simulink library "tqr"  (R2021b)
settings: Solver=VariableStepAuto  StartTime=0.0  StopTime=10.0  RelTol=1e-3
undefined symbols (not defined in the file or in its folder): ATQR_AltRDCActiveFEDUInc_X_pct, ATQR_AltRDCActiveFEDUInc_Y_enum, ATQR_AltRDCActiveFEDUTs_X_pct, ATQR_AltRDCActiveFEDUTs_Y_enum, ATQR_AltRDCActiveREDUInc_X_pct, ATQR_AltRDCActiveREDUInc_Y_enum, ATQR_AltRDCActiveREDUTs_X_pct, ATQR_AltRDCActiveREDUTs_Y_enum, ATQR_CreepFEDUTqIncSR_X_rpm, ATQR_CreepFEDUTqIncSR_Y_Nm, ATQR_CreepFEDUTs_X_rpm, ATQR_CreepFEDUTs_Y_Nm, ATQR_EcoTqFrIncGain_X_Nm, ATQR_EcoTqFrIncGain_Y_pct, ATQR_EcoTqRrIncGain_X_Nm, ATQR_EcoTqRrIncGain_Y_pct, ATQR_EL1FEDUTqDecSR_Y_Nm, ATQR_EL1FEDUTqIncSR_X_rpm, ATQR_EL1FEDUTqIncSR_Y_pct, ATQR_EL1FEDUTs_X_rpm, ATQR_EL1FEDUTs_Y_Nm, ATQR_EL1REDUTqDecSR_Y_Nm, ATQR_EL1REDUTs_Y_Nm, ATQR_FEDUEL1RegenTs_X_rpm, ATQR_FEDUTIPOutTs_X_rpm, ATQR_FrNegRateLimitIncN_X_rpm, ATQR_FrNegRateLimitIncN_Y_Nm, ATQR_FrPosRateLimitIncN_X_rpm, ATQR_FrPosRateLimitIncN_Y_Nm, ATQR_FShaftSpdTqLimCoe_X_rpm, ATQR_FTimerTqLimCoe_X_s, ATQR_FTqZeroTransUpBoundN_X_rpm, ATQR_NL1FEDUTqDecSR_Y_Nm, ATQR_NL1FEDUTqIncSR_X_rpm, ATQR_NL1FEDUTqIncSR_Y_pct, ATQR_NL1FEDUTs_X_rpm, ATQR_NL1FEDUTs_Y_Nm, ATQR_NL1REDUTqDecSR_Y_Nm, ATQR_NL1REDUTs_Y_Nm, ATQR_NormalTqFrIncGain_X_Nm, ATQR_NormalTqFrIncGain_Y_pct, ATQR_NormalTqRrIncGain_X_Nm, ATQR_NormalTqRrIncGain_Y_pct, ATQR_RrNegRateLimitIncN_X_rpm, ATQR_RrNegRateLimitIncN_Y_Nm, ATQR_RrPosRateLimitIncN_X_rpm, ATQR_RrPosRateLimitIncN_Y_Nm, ATQR_RShaftSpdTqLimCoe_X_rpm, ATQR_RTimerTqLimCoe_X_s, ATQR_SL1FEDUTqDecSR_Y_Nm, ATQR_SL1FEDUTqIncSR_X_rpm, ATQR_SL1FEDUTqIncSR_Y_pct, ATQR_SL1FEDUTs_X_rpm, ATQR_SL1FEDUTs_Y_Nm, ATQR_SL1REDUTqDecSR_Y_Nm, ATQR_SL1REDUTs_Y_Nm, ATQR_SportTqFrIncGain_X_Nm, ATQR_SportTqFrIncGain_Y_pct, ATQR_SportTqRrIncGain_X_Nm, ATQR_SportTqRrIncGain_Y_pct ... (+261)
libraries: hcu_lib x14, simulink x12, $bdroot x3
(part 5 of 9)

== system tqr/TQR/Determine Torque Request/TorqueArbitrament/TorqueSmooth/Front wheel rate limit determination/Negative Rate limit Determination ==
  VTQD_TqTargetShaftSpd_rpm : Inport
  VTQR_FEDUWhlTqReqSmoothDelay_Nm : Inport  Port=2
  VTQR_EVDriveMode_enum : Inport  Port=3
  Constant1 : Constant  Value=ENUM_DRIVEMODE_ECO
  Constant2 : Constant  Value=ENUM_DRIVEMODE_NRM
  Constant3 : Constant  Value=ENUM_DRIVEMODE_SPORT
  Constant7 : Constant  Value=ENUM_DRIVEMODE_ECO
  Constant8 : Constant  Value=ENUM_DRIVEMODE_NRM
  Constant9 : Constant  Value=ENUM_DRIVEMODE_SPORT
  Equal{1..3,5..6,8} (6 alike) : RelationalOperator  Operator===  OutDataTypeStr=boolean  RndMeth=Simplest
  If1 : If  NumInputs=3  IfExpression=u1~= 0  ElseIfExpressions=u2 ~= 0, u3 ~= 0  ShowElse=off
  If2 : If  NumInputs=3  IfExpression=u1~= 0  ElseIfExpressions=u2 ~= 0, u3 ~= 0  ShowElse=off
  Merge1 : Merge  Inputs=3
  Merge2 : Merge  Inputs=3
  Mux : Mux  Inputs=2
  VTQR_FrNegRateLimitDecE_Nm : Subsystem  TreatAsAtomicUnit=on
  VTQR_FrNegRateLimitDecN_Nm : Subsystem  TreatAsAtomicUnit=on
  VTQR_FrNegRateLimitDecS_Nm : Subsystem  TreatAsAtomicUnit=on
  VTQR_FrNegRateLimitIncE_Nm : Subsystem  TreatAsAtomicUnit=on
  VTQR_FrNegRateLimitIncN_Nm : Subsystem  TreatAsAtomicUnit=on
  VTQR_FrNegRateLimitIncS_Nm : Subsystem  TreatAsAtomicUnit=on
  VTQR_NegRateLimit_mux : Outport
  wires:
  Merge2/1 -> Mux/2  "VTQR_NegRateLimitDec_Nm"
  Constant1/1 -> Equal1/2
  [VTQD_TqTargetShaftSpd_rpm] -> VTQR_FrNegRateLimitDecE_Nm/1(VTQD_TqTargetShaftSpd_rpm)
  [VTQR_FEDUWhlTqReqSmoothDelay_Nm] -> VTQR_FrNegRateLimitDecN_Nm/2(VTQR_FEDUWhlTqReqSmoothDelay_Nm)
  [VTQD_TqTargetShaftSpd_rpm] -> VTQR_FrNegRateLimitDecN_Nm/1(VTQD_TqTargetShaftSpd_rpm)
  [VTQR_EVDriveMode_enum] -> Equal1/1
  Equal2/1 -> If2/1
  Constant2/1 -> Equal2/2
  Constant3/1 -> Equal3/2
  Equal3/1 -> If2/3
  If2/2 -> VTQR_FrNegRateLimitDecE_Nm/Action
  [VTQR_EVDriveMode_enum] -> Equal3/1
  [VTQR_EVDriveMode_enum] -> Equal2/1
  VTQR_FrNegRateLimitDecE_Nm/1(VTQR_FrNegRateLimitDecE_Nm) -> Merge2/2
  [VTQR_FEDUWhlTqReqSmoothDelay_Nm] -> VTQR_FrNegRateLimitDecE_Nm/2(VTQR_FEDUWhlTqReqSmoothDelay_Nm)
  If2/1 -> VTQR_FrNegRateLimitDecN_Nm/Action
  [VTQR_FEDUWhlTqReqSmoothDelay_Nm] -> VTQR_FrNegRateLimitDecS_Nm/2(VTQR_FEDUWhlTqReqSmoothDelay_Nm)
  [VTQD_TqTargetShaftSpd_rpm] -> VTQR_FrNegRateLimitDecS_Nm/1(VTQD_TqTargetShaftSpd_rpm)
  VTQR_FrNegRateLimitDecS_Nm/1(VTQR_FrNegRateLimitDecS_Nm) -> Merge2/3
  Equal1/1 -> If2/2
  If2/3 -> VTQR_FrNegRateLimitDecS_Nm/Action
  VTQR_FrNegRateLimitDecN_Nm/1(VTQR_FrNegRateLimitDecN_Nm) -> Merge2/1
  VTQR_FrNegRateLimitIncE_Nm/1(VTQR_FrNegRateLimitIncE_Nm) -> Merge1/2
  VTQR_FrNegRateLimitIncS_Nm/1(VTQR_FrNegRateLimitIncS_Nm) -> Merge1/3
  If1/2 -> VTQR_FrNegRateLimitIncE_Nm/Action
  If1/3 -> VTQR_FrNegRateLimitIncS_Nm/Action
  [VTQD_TqTargetShaftSpd_rpm] -> VTQR_FrNegRateLimitIncS_Nm/1(VTQD_TqTargetShaftSpd_rpm)
  [VTQR_FEDUWhlTqReqSmoothDelay_Nm] -> VTQR_FrNegRateLimitIncS_Nm/2(VTQR_FEDUWhlTqReqSmoothDelay_Nm)
  [VTQR_FEDUWhlTqReqSmoothDelay_Nm] -> VTQR_FrNegRateLimitIncE_Nm/2(VTQR_FEDUWhlTqReqSmoothDelay_Nm)
  [VTQD_TqTargetShaftSpd_rpm] -> VTQR_FrNegRateLimitIncE_Nm/1(VTQD_TqTargetShaftSpd_rpm)
  VTQR_FrNegRateLimitIncN_Nm/1(VTQR_FrNegRateLimitIncN_Nm) -> Merge1/1
  If1/1 -> VTQR_FrNegRateLimitIncN_Nm/Action
  [VTQR_FEDUWhlTqReqSmoothDelay_Nm] -> VTQR_FrNegRateLimitIncN_Nm/2(VTQR_FEDUWhlTqReqSmoothDelay_Nm)
  [VTQD_TqTargetShaftSpd_rpm] -> VTQR_FrNegRateLimitIncN_Nm/1(VTQD_TqTargetShaftSpd_rpm)
  Equal8/1 -> If1/3
  Equal5/1 -> If1/2
  Equal6/1 -> If1/1
  [VTQR_EVDriveMode_enum] -> Equal6/1
  [VTQR_EVDriveMode_enum] -> Equal8/1
  [VTQR_EVDriveMode_enum] -> Equal5/1
  Constant8/1 -> Equal6/2
  Constant9/1 -> Equal8/2
  Constant7/1 -> Equal5/2
  Merge1/1 -> Mux/1  "VTQR_NegRateLimitInc_Nm"
  Mux/1 -> VTQR_NegRateLimit_mux/1  "VTQR_NegRateLimit_mux"
  VTQD_TqTargetShaftSpd_rpm/1 -> [VTQD_TqTargetShaftSpd_rpm]
  VTQR_FEDUWhlTqReqSmoothDelay_Nm/1 -> [VTQR_FEDUWhlTqReqSmoothDelay_Nm]
  VTQR_EVDriveMode_enum/1 -> [VTQR_EVDriveMode_enum]

== system tqr/TQR/Determine Torque Request/TorqueArbitrament/TorqueSmooth/Front wheel rate limit determination/Positive Rate limit Determination ==
  VTQD_TqTargetShaftSpd_rpm : Inport
  VTQR_FEDUWhlTqReqSmoothDelay_Nm : Inport  Port=2
  VTQR_EVDriveMode_enum : Inport  Port=3
  Constant1 : Constant  Value=ENUM_DRIVEMODE_ECO
  Constant2 : Constant  Value=ENUM_DRIVEMODE_NRM
  Constant3 : Constant  Value=ENUM_DRIVEMODE_SPORT
  Constant7 : Constant  Value=ENUM_DRIVEMODE_ECO
  Constant8 : Constant  Value=ENUM_DRIVEMODE_NRM
  Constant9 : Constant  Value=ENUM_DRIVEMODE_SPORT
  Equal{1..3,5..6,8} (6 alike) : RelationalOperator  Operator===  OutDataTypeStr=boolean  RndMeth=Simplest
  If1 : If  NumInputs=3  IfExpression=u1~= 0  ElseIfExpressions=u2 ~= 0, u3 ~= 0  ShowElse=off
  If2 : If  NumInputs=3  IfExpression=u1~= 0  ElseIfExpressions=u2 ~= 0, u3 ~= 0  ShowElse=off
  Merge1 : Merge  Inputs=3
  Merge2 : Merge  Inputs=3
  Mux : Mux  Inputs=2
  VTQR_FrPosRateLimitDecE_Nm : Subsystem  TreatAsAtomicUnit=on
  VTQR_FrPosRateLimitDecN_Nm : Subsystem  TreatAsAtomicUnit=on
  VTQR_FrPosRateLimitDecS_Nm : Subsystem  TreatAsAtomicUnit=on
  VTQR_FrPosRateLimitIncE_Nm : Subsystem  TreatAsAtomicUnit=on
  VTQR_FrPosRateLimitIncN_Nm : Subsystem  TreatAsAtomicUnit=on
  VTQR_FrPosRateLimitIncS_Nm : Subsystem  TreatAsAtomicUnit=on
  VTQR_PosRateLimit_mux : Outport
  wires:
  VTQD_TqTargetShaftSpd_rpm/1 -> [VTQD_TqTargetShaftSpd_rpm]
  Mux/1 -> VTQR_PosRateLimit_mux/1  "VTQR_PosRateLimit_mux"
  Merge1/1 -> Mux/1  "VTQR_PosRateLimitInc_Nm"
  Constant7/1 -> Equal5/2
  Constant9/1 -> Equal8/2
  Constant8/1 -> Equal6/2
  [VTQR_EVDriveMode_enum] -> Equal5/1
  [VTQR_EVDriveMode_enum] -> Equal8/1
  [VTQR_EVDriveMode_enum] -> Equal6/1
  Equal6/1 -> If1/1
  Equal5/1 -> If1/2
  Equal8/1 -> If1/3
  [VTQD_TqTargetShaftSpd_rpm] -> VTQR_FrPosRateLimitIncN_Nm/1(VTQD_TqTargetShaftSpd_rpm)
  [VTQR_FEDUWhlTqReqSmoothDelay_Nm] -> VTQR_FrPosRateLimitIncN_Nm/2(VTQR_FEDUWhlTqReqSmoothDelay_Nm)
  If1/1 -> VTQR_FrPosRateLimitIncN_Nm/Action
  VTQR_FrPosRateLimitIncN_Nm/1(VTQR_FrPosRateLimitIncN_Nm) -> Merge1/1
  [VTQD_TqTargetShaftSpd_rpm] -> VTQR_FrPosRateLimitIncE_Nm/1(VTQD_TqTargetShaftSpd_rpm)
  [VTQR_FEDUWhlTqReqSmoothDelay_Nm] -> VTQR_FrPosRateLimitIncE_Nm/2(VTQR_FEDUWhlTqReqSmoothDelay_Nm)
  [VTQR_FEDUWhlTqReqSmoothDelay_Nm] -> VTQR_FrPosRateLimitIncS_Nm/2(VTQR_FEDUWhlTqReqSmoothDelay_Nm)
  [VTQD_TqTargetShaftSpd_rpm] -> VTQR_FrPosRateLimitIncS_Nm/1(VTQD_TqTargetShaftSpd_rpm)
  If1/3 -> VTQR_FrPosRateLimitIncS_Nm/Action
  If1/2 -> VTQR_FrPosRateLimitIncE_Nm/Action
  VTQR_FrPosRateLimitIncS_Nm/1(VTQR_FrPosRateLimitIncS_Nm) -> Merge1/3
  VTQR_FrPosRateLimitIncE_Nm/1(VTQR_FrPosRateLimitIncE_Nm) -> Merge1/2
  VTQR_FrPosRateLimitDecN_Nm/1(VTQR_FrPosRateLimitDecN_Nm) -> Merge2/1
  If2/3 -> VTQR_FrPosRateLimitDecS_Nm/Action
  Equal1/1 -> If2/2
  VTQR_FrPosRateLimitDecS_Nm/1(VTQR_FrPosRateLimitDecS_Nm) -> Merge2/3
  [VTQD_TqTargetShaftSpd_rpm] -> VTQR_FrPosRateLimitDecS_Nm/1(VTQD_TqTargetShaftSpd_rpm)
  [VTQR_FEDUWhlTqReqSmoothDelay_Nm] -> VTQR_FrPosRateLimitDecS_Nm/2(VTQR_FEDUWhlTqReqSmoothDelay_Nm)
  If2/1 -> VTQR_FrPosRateLimitDecN_Nm/Action
  [VTQR_FEDUWhlTqReqSmoothDelay_Nm] -> VTQR_FrPosRateLimitDecE_Nm/2(VTQR_FEDUWhlTqReqSmoothDelay_Nm)
  VTQR_FrPosRateLimitDecE_Nm/1(VTQR_FrPosRateLimitDecE_Nm) -> Merge2/2
  [VTQR_EVDriveMode_enum] -> Equal2/1
  [VTQR_EVDriveMode_enum] -> Equal3/1
  If2/2 -> VTQR_FrPosRateLimitDecE_Nm/Action
  Equal3/1 -> If2/3
  Constant3/1 -> Equal3/2
  Constant2/1 -> Equal2/2
  Equal2/1 -> If2/1
  [VTQR_EVDriveMode_enum] -> Equal1/1
  [VTQD_TqTargetShaftSpd_rpm] -> VTQR_FrPosRateLimitDecN_Nm/1(VTQD_TqTargetShaftSpd_rpm)
  [VTQR_FEDUWhlTqReqSmoothDelay_Nm] -> VTQR_FrPosRateLimitDecN_Nm/2(VTQR_FEDUWhlTqReqSmoothDelay_Nm)
  [VTQD_TqTargetShaftSpd_rpm] -> VTQR_FrPosRateLimitDecE_Nm/1(VTQD_TqTargetShaftSpd_rpm)
  Constant1/1 -> Equal1/2
  Merge2/1 -> Mux/2  "VTQR_PosRateLimitDec_Nm"
  VTQR_FEDUWhlTqReqSmoothDelay_Nm/1 -> [VTQR_FEDUWhlTqReqSmoothDelay_Nm]
  VTQR_EVDriveMode_enum/1 -> [VTQR_EVDriveMode_enum]

== system tqr/TQR/Determine Torque Request/TorqueArbitrament/TorqueSmooth/Front wheel rate limit determination/VTQR_ECOFEDURateLimitDec_Nm ==
  VTQR_FEDUWhlTqReqSmoothDelay_Nm : Inport
  VTQD_TqTargetShaftSpd_rpm : Inport  Port=2
  VTQD_RegenMode_enum : Inport  Port=3
  Action Port : ActionPort
  Constant : Constant  Value=ENUM_REGENLEVEL_LV1
  Constant1 : Constant  Value=ENUM_REGENLEVEL_LV2
  Constant2 : Constant  Value=ENUM_REGENLEVEL_LV3
  Constant3 : Constant  Value=ENUM_REGENLEVEL_LV4
  Constant4 : Constant  Value=ENUM_REGENLEVEL_LV5
  Constant5 : Constant  Value=ENUM_REGENLEVEL_OPD
  Equal{,1..5} (6 alike) : RelationalOperator  Operator===  OutDataTypeStr=boolean  RndMeth=Simplest
  If : If  NumInputs=6  IfExpression=u1~= 0  ElseIfExpressions=u2 ~= 0, u3 ~= 0,u4 ~= 0,u5~=0,u6~=0
  Invalid : Subsystem  TreatAsAtomicUnit=on
  LV1 : Subsystem  TreatAsAtomicUnit=on
  LV2 : Subsystem  AncestorBlock=tqr/TQR/Determine Torque Request/TorqueArbitrament/TorqueSmooth/Front First order filter input tau map and determination/VTQR_ECOFEDUTs_c/LV2  TreatAsAtomicUnit=on
  LV3 : Subsystem  AncestorBlock=tqr/TQR/Determine Torque Request/TorqueArbitrament/TorqueSmooth/Front First order filter input tau map and determination/VTQR_ECOFEDUTs_c/LV3  TreatAsAtomicUnit=on
  LV4 : Subsystem  AncestorBlock=tqr/TQR/Determine Torque Request/TorqueArbitrament/TorqueSmooth/Front First order filter input tau map and determination/VTQR_ECOFEDUTs_c/LV4  TreatAsAtomicUnit=on
  LV5 : Subsystem  AncestorBlock=tqr/TQR/Determine Torque Request/TorqueArbitrament/TorqueSmooth/Front First order filter input tau map and determination/VTQR_ECOFEDUTs_c/LV5  TreatAsAtomicUnit=on
  Merge : Merge  Inputs=7
  OPD : Subsystem  AncestorBlock=tqr/TQR/Determine Torque Request/TorqueArbitrament/TorqueSmooth/Front First order filter input tau map and determination/VTQR_ECOFEDUTs_c/OPD  TreatAsAtomicUnit=on
  VTQR_ECOFEDURateLimitDec_Nm : Outport
  wires:
  [VTQD_TqTargetShaftSpd_rpm] -> LV2/2(VTQD_TqTargetShaftSpd_rpm)
  Constant3/1 -> Equal3/2
  If/3 -> LV3/Action
  Equal2/1 -> If/3
  Constant4/1 -> Equal4/2
  Constant/1 -> Equal/2
  Equal5/1 -> If/6
  OPD/1(VTQR_EOPDFEDUTqDecSR_Nm) -> Merge/6
  [VTQD_RegenMode_enum] -> Equal4/1
  [VTQR_FEDUWhlTqReqSmoothDelay_Nm] -> LV2/1(VTQR_FEDUWhlTqReqSmoothDelay_Nm)
  LV2/1(VTQR_EL2FEDUTqDecSR_Nm) -> Merge/2
  [VTQD_RegenMode_enum] -> Equal5/1
  [VTQR_FEDUWhlTqReqSmoothDelay_Nm] -> OPD/1(VTQR_FEDUWhlTqReqSmoothDelay_Nm)
  [VTQD_RegenMode_enum] -> Equal2/1
  [VTQD_TqTargetShaftSpd_rpm] -> LV1/2(VTQD_TqTargetShaftSpd_rpm)
  [VTQR_FEDUWhlTqReqSmoothDelay_Nm] -> LV5/1(VTQR_FEDUWhlTqReqSmoothDelay_Nm)
  [VTQD_TqTargetShaftSpd_rpm] -> OPD/2(VTQD_TqTargetShaftSpd_rpm)
  [VTQD_TqTargetShaftSpd_rpm] -> LV4/2(VTQD_TqTargetShaftSpd_rpm)
  [VTQR_FEDUWhlTqReqSmoothDelay_Nm] -> LV3/1(VTQR_FEDUWhlTqReqSmoothDelay_Nm)
  Constant5/1 -> Equal5/2
  [VTQR_FEDUWhlTqReqSmoothDelay_Nm] -> LV4/1(VTQR_FEDUWhlTqReqSmoothDelay_Nm)
  [VTQD_TqTargetShaftSpd_rpm] -> LV5/2(VTQD_TqTargetShaftSpd_rpm)
  Equal/1 -> If/1
  If/2 -> LV2/Action
  If/4 -> LV4/Action
  Constant1/1 -> Equal1/2
  LV1/1(VTQR_EL1FEDUTqDecSR_Nm) -> Merge/1
  [VTQD_RegenMode_enum] -> Equal/1
  Equal4/1 -> If/5
  Equal1/1 -> If/2
  If/6 -> OPD/Action
  [VTQD_RegenMode_enum] -> Equal3/1
  LV3/1(VTQR_EL3FEDUTqDecSR_Nm) -> Merge/3
  LV5/1(VTQR_EL5FEDUTqIDecSR_Nm) -> Merge/5
  [VTQD_RegenMode_enum] -> Equal1/1
  Equal3/1 -> If/4
  LV4/1(VTQR_EL4FEDUTqDecSR_Nm) -> Merge/4
  [VTQD_TqTargetShaftSpd_rpm] -> LV3/2(VTQD_TqTargetShaftSpd_rpm)
  [VTQR_FEDUWhlTqReqSmoothDelay_Nm] -> LV1/1(VTQR_FEDUWhlTqReqSmoothDelay_Nm)
  If/5 -> LV5/Action
  If/1 -> LV1/Action
  Constant2/1 -> Equal2/2
  Merge/1 -> VTQR_ECOFEDURateLimitDec_Nm/1  "VTQR_ECOFEDURateLimitDec_Nm"
  VTQR_FEDUWhlTqReqSmoothDelay_Nm/1 -> [VTQR_FEDUWhlTqReqSmoothDelay_Nm]
  VTQD_TqTargetShaftSpd_rpm/1 -> [VTQD_TqTargetShaftSpd_rpm]
  VTQD_RegenMode_enum/1 -> [VTQD_RegenMode_enum]
  [VTQR_FEDUWhlTqReqSmoothDelay_Nm] -> Invalid/1(VTQR_FEDUWhlTqReqSmoothDelay_Nm)
  [VTQD_TqTargetShaftSpd_rpm] -> Invalid/2(VTQD_TqTargetShaftSpd_rpm)
  If/7 -> Invalid/Action
  Invalid/1(VTQR_EL1FEDUTqDecSR_Nm) -> Merge/7

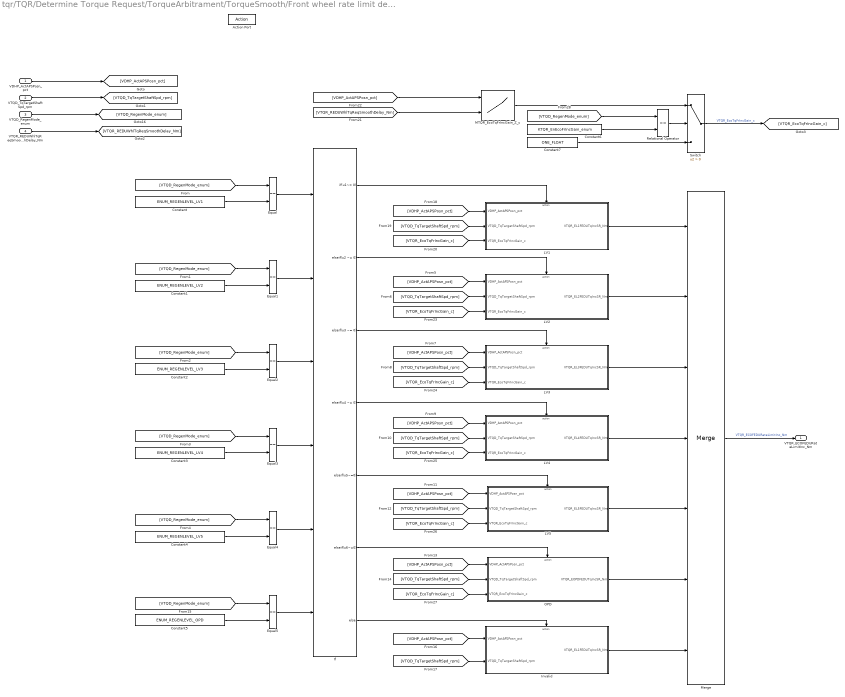
== system tqr/TQR/Determine Torque Request/TorqueArbitrament/TorqueSmooth/Front wheel rate limit determination/VTQR_ECOFEDURateLimitInc_Nm ==
  VDHP_ActAPSPosn_pct : Inport
  VTQD_TqTargetShaftSpd_rpm : Inport  Port=2
  VTQD_RegenMode_enum : Inport  Port=3
  VTQR_REDUWhlTqReqSmoothDelay_Nm : Inport  Port=4
  Action Port : ActionPort
  Constant : Constant  Value=ENUM_REGENLEVEL_LV1
  Constant1 : Constant  Value=ENUM_REGENLEVEL_LV2
  Constant2 : Constant  Value=ENUM_REGENLEVEL_LV3
  Constant3 : Constant  Value=ENUM_REGENLEVEL_LV4
  Constant4 : Constant  Value=ENUM_REGENLEVEL_LV5
  Constant5 : Constant  Value=ENUM_REGENLEVEL_OPD
  Constant6 : Constant  Value=KTQR_EnEcoFrIncGain_enum
  Constant7 : Constant  Value=ONE_FLOAT
  Equal{,1..5} (6 alike) : RelationalOperator  Operator===  OutDataTypeStr=boolean  RndMeth=Simplest
  If : If  NumInputs=6  IfExpression=u1~= 0  ElseIfExpressions=u2 ~= 0, u3 ~= 0,u4 ~= 0,u5~=0,u6~=0
  Invalid : Subsystem  TreatAsAtomicUnit=on
  LV1 : Subsystem  TreatAsAtomicUnit=on
  LV2 : Subsystem  TreatAsAtomicUnit=on
  LV3 : Subsystem  TreatAsAtomicUnit=on
  LV4 : Subsystem  TreatAsAtomicUnit=on
  LV5 : Subsystem  TreatAsAtomicUnit=on
  MTQR_EcoTqFrIncGain_Z_c : Lookup_n-D  BreakpointsForDimension1=ATQR_EcoTqFrIncGain_Y_pct  BreakpointsForDimension2=ATQR_EcoTqFrIncGain_X_Nm  Table=MTQR_EcoTqFrIncGain_Z_c  ExtrapMethod=Clip  InternalRulePriority=Speed  RndMeth=Simplest  InputSameDT=on
      settings: InputPortMap=u0,u1
  Merge : Merge  Inputs=7
  OPD : Subsystem  TreatAsAtomicUnit=on
  Relational Operator : RelationalOperator  OutDataTypeStr=boolean  RndMeth=Simplest
  Switch : Switch  Criteria=u2 > Threshold
  VTQR_ECOFEDURateLimitInc_Nm : Outport
  wires:
  [VTQD_TqTargetShaftSpd_rpm] -> LV2/2(VTQD_TqTargetShaftSpd_rpm)
  Constant3/1 -> Equal3/2
  If/3 -> LV3/Action
  Equal2/1 -> If/3
  Constant4/1 -> Equal4/2
  Constant/1 -> Equal/2
  Equal5/1 -> If/6
  OPD/1(VTQR_EOPDFEDUTqIncSR_Nm) -> Merge/6
  [VTQD_RegenMode_enum] -> Equal4/1
  [VDHP_ActAPSPosn_pct] -> LV2/1(VDHP_ActAPSPosn_pct)
  LV2/1(VTQR_EL2FEDUTqIncSR_Nm) -> Merge/2
  [VTQD_RegenMode_enum] -> Equal5/1
  [VDHP_ActAPSPosn_pct] -> OPD/1(VDHP_ActAPSPosn_pct)
  [VTQD_RegenMode_enum] -> Equal2/1
  [VTQD_TqTargetShaftSpd_rpm] -> LV1/2(VTQD_TqTargetShaftSpd_rpm)
  [VDHP_ActAPSPosn_pct] -> LV5/1(VDHP_ActAPSPosn_pct)
  [VTQD_TqTargetShaftSpd_rpm] -> OPD/2(VTQD_TqTargetShaftSpd_rpm)
  [VTQD_TqTargetShaftSpd_rpm] -> LV4/2(VTQD_TqTargetShaftSpd_rpm)
  [VDHP_ActAPSPosn_pct] -> LV3/1(VDHP_ActAPSPosn_pct)
  Constant5/1 -> Equal5/2
  [VDHP_ActAPSPosn_pct] -> LV4/1(VDHP_ActAPSPosn_pct)
  [VTQD_TqTargetShaftSpd_rpm] -> LV5/2(VTQD_TqTargetShaftSpd_rpm)
  Equal/1 -> If/1
  If/2 -> LV2/Action
  If/4 -> LV4/Action
  Constant1/1 -> Equal1/2
  LV1/1(VTQR_EL1FEDUTqIncSR_Nm) -> Merge/1
  [VTQD_RegenMode_enum] -> Equal/1
  Equal4/1 -> If/5
  Equal1/1 -> If/2
  If/6 -> OPD/Action
  [VTQD_RegenMode_enum] -> Equal3/1
  LV3/1(VTQR_EL3FEDUTqIncSR_Nm) -> Merge/3
  LV5/1(VTQR_EL5FEDUTqIncSR_Nm) -> Merge/5
  [VTQD_RegenMode_enum] -> Equal1/1
  Equal3/1 -> If/4
  LV4/1(VTQR_EL4FEDUTqIncSR_Nm) -> Merge/4
  [VTQD_TqTargetShaftSpd_rpm] -> LV3/2(VTQD_TqTargetShaftSpd_rpm)
  [VDHP_ActAPSPosn_pct] -> LV1/1(VDHP_ActAPSPosn_pct)
  If/5 -> LV5/Action
  If/1 -> LV1/Action
  Constant2/1 -> Equal2/2
  Merge/1 -> VTQR_ECOFEDURateLimitInc_Nm/1  "VTQR_ECOFEDURateLimitInc_Nm"
  VDHP_ActAPSPosn_pct/1 -> [VDHP_ActAPSPosn_pct]
  VTQD_TqTargetShaftSpd_rpm/1 -> [VTQD_TqTargetShaftSpd_rpm]
  VTQD_RegenMode_enum/1 -> [VTQD_RegenMode_enum]
  [VDHP_ActAPSPosn_pct] -> Invalid/1(VDHP_ActAPSPosn_pct)
  [VTQD_TqTargetShaftSpd_rpm] -> Invalid/2(VTQD_TqTargetShaftSpd_rpm)
  If/7 -> Invalid/Action
  Invalid/1(VTQR_EL1FEDUTqIncSR_Nm) -> Merge/7
  [VDHP_ActAPSPosn_pct] -> MTQR_EcoTqFrIncGain_Z_c/1
  [VTQR_EcoTqFrIncGain_c] -> LV1/3(VTQR_EcoTqFrIncGain_c)
  [VTQR_EcoTqFrIncGain_c] -> LV2/3(VTQR_EcoTqFrIncGain_c)
  [VTQR_EcoTqFrIncGain_c] -> LV3/3(VTQR_EcoTqFrIncGain_c)
  [VTQR_EcoTqFrIncGain_c] -> LV4/3(VTQR_EcoTqFrIncGain_c)
  [VTQR_EcoTqFrIncGain_c] -> LV5/3(VTQR_EcoTqFrIncGain_c)
  [VTQR_EcoTqFrIncGain_c] -> OPD/3(VTQR_EcoTqFrIncGain_c)
  VTQR_REDUWhlTqReqSmoothDelay_Nm/1 -> [VTQR_REDUWhlTqReqSmoothDelay_Nm]
  [VTQR_REDUWhlTqReqSmoothDelay_Nm] -> MTQR_EcoTqFrIncGain_Z_c/2
  Relational Operator/1 -> Switch/2
  Constant6/1 -> Relational Operator/2
  [VTQD_RegenMode_enum] -> Relational Operator/1
  Constant7/1 -> Switch/3
  MTQR_EcoTqFrIncGain_Z_c/1 -> Switch/1
  Switch/1 -> [VTQR_EcoTqFrIncGain_c]  "VTQR_EcoTqFrIncGain_c"

== system tqr/TQR/Determine Torque Request/TorqueArbitrament/TorqueSmooth/Front wheel rate limit determination/VTQR_LHMFEDURateLimitDec_Nm ==
  VTQR_FEDUWhlTqReqSmoothDelay_Nm : Inport
  VTQD_TqTargetShaftSpd_rpm : Inport  Port=2
  Action Port : ActionPort
  MTQR_LHMFEDUTqDecSR_Z_Nm : Lookup_n-D  BreakpointsForDimension1=ATQR_NL1FEDUTqDecSR_Y_Nm  BreakpointsForDimension2=ATQR_NL1FEDUTqIncSR_X_rpm  Table=MTQR_LHMFEDUTqDecSR_Z_Nm  ExtrapMethod=Clip  InternalRulePriority=Speed  RndMeth=Simplest  InputSameDT=on
      settings: InputPortMap=u0,u1
  VTQR_LHMFEDURateLimitDec_Nm : Outport
  wires:
  VTQR_FEDUWhlTqReqSmoothDelay_Nm/1 -> MTQR_LHMFEDUTqDecSR_Z_Nm/1
  VTQD_TqTargetShaftSpd_rpm/1 -> MTQR_LHMFEDUTqDecSR_Z_Nm/2
  MTQR_LHMFEDUTqDecSR_Z_Nm/1 -> VTQR_LHMFEDURateLimitDec_Nm/1  "VTQR_LHMFEDURateLimitDec_Nm"

== system tqr/TQR/Determine Torque Request/TorqueArbitrament/TorqueSmooth/Front wheel rate limit determination/VTQR_LHMFEDURateLimitInc_Nm ==
  VDHP_ActAPSPosn_pct : Inport
  VTQD_TqTargetShaftSpd_rpm : Inport  Port=2
  Action Port : ActionPort
  MTQR_LHMFEDUTqIncSR_Z_Nm : Lookup_n-D  BreakpointsForDimension1=ATQR_NL1FEDUTqIncSR_Y_pct  BreakpointsForDimension2=ATQR_NL1FEDUTqIncSR_X_rpm  Table=MTQR_LHMFEDUTqIncSR_Z_Nm  ExtrapMethod=Clip  InternalRulePriority=Speed  RndMeth=Simplest  InputSameDT=on
      settings: InputPortMap=u0,u1
  VTQR_LHMFEDURateLimitInc_Nm : Outport
  wires:
  VDHP_ActAPSPosn_pct/1 -> MTQR_LHMFEDUTqIncSR_Z_Nm/1
  VTQD_TqTargetShaftSpd_rpm/1 -> MTQR_LHMFEDUTqIncSR_Z_Nm/2
  MTQR_LHMFEDUTqIncSR_Z_Nm/1 -> VTQR_LHMFEDURateLimitInc_Nm/1  "VTQR_LHMFEDURateLimitInc_Nm"

== system tqr/TQR/Determine Torque Request/TorqueArbitrament/TorqueSmooth/Front wheel rate limit determination/VTQR_NORMALFEDURateLimitDec_Nm ==
  VTQR_FEDUWhlTqReqSmoothDelay_Nm : Inport
  VTQD_TqTargetShaftSpd_rpm : Inport  Port=2
  VTQD_RegenMode_enum : Inport  Port=3
  Action Port : ActionPort
  Constant : Constant  Value=ENUM_REGENLEVEL_LV1
  Constant1 : Constant  Value=ENUM_REGENLEVEL_LV2
  Constant2 : Constant  Value=ENUM_REGENLEVEL_LV3
  Constant3 : Constant  Value=ENUM_REGENLEVEL_LV4
  Constant4 : Constant  Value=ENUM_REGENLEVEL_LV5
  Constant5 : Constant  Value=ENUM_REGENLEVEL_OPD
  Equal{,1..5} (6 alike) : RelationalOperator  Operator===  OutDataTypeStr=boolean  RndMeth=Simplest
  If : If  NumInputs=6  IfExpression=u1~= 0  ElseIfExpressions=u2 ~= 0, u3 ~= 0,u4 ~= 0,u5~=0,u6~=0
  Invalid : Subsystem  TreatAsAtomicUnit=on
  LV1 : Subsystem  AncestorBlock=tqr/TQR/Determine Torque Request/TorqueArbitrament/TorqueSmooth/Front wheel rate limit determination/VTQR_ECOFEDURateLimitDec_Nm/LV1  TreatAsAtomicUnit=on
  LV2 : Subsystem  AncestorBlock=tqr/TQR/Determine Torque Request/TorqueArbitrament/TorqueSmooth/Front wheel rate limit determination/VTQR_ECOFEDURateLimitDec_Nm/LV2  TreatAsAtomicUnit=on
  LV3 : Subsystem  AncestorBlock=tqr/TQR/Determine Torque Request/TorqueArbitrament/TorqueSmooth/Front wheel rate limit determination/VTQR_ECOFEDURateLimitDec_Nm/LV3  TreatAsAtomicUnit=on
  LV4 : Subsystem  AncestorBlock=tqr/TQR/Determine Torque Request/TorqueArbitrament/TorqueSmooth/Front wheel rate limit determination/VTQR_ECOFEDURateLimitDec_Nm/LV4  TreatAsAtomicUnit=on
  LV5 : Subsystem  AncestorBlock=tqr/TQR/Determine Torque Request/TorqueArbitrament/TorqueSmooth/Front wheel rate limit determination/VTQR_ECOFEDURateLimitDec_Nm/LV5  TreatAsAtomicUnit=on
  Merge : Merge  Inputs=7
  OPD : Subsystem  AncestorBlock=tqr/TQR/Determine Torque Request/TorqueArbitrament/TorqueSmooth/Front wheel rate limit determination/VTQR_ECOFEDURateLimitDec_Nm/OPD  TreatAsAtomicUnit=on
  VTQR_NORMALFEDURateLimitDec_Nm : Outport
  wires:
  Equal2/1 -> If/3
  [VTQD_TqTargetShaftSpd_rpm] -> LV2/2(VTQD_TqTargetShaftSpd_rpm)
  Constant3/1 -> Equal3/2
  OPD/1(VTQR_NOPDFEDUTqDecSR_Nm) -> Merge/6
  If/3 -> LV3/Action
  Equal5/1 -> If/6
  [VTQD_RegenMode_enum] -> Equal4/1
  LV5/1(VTQR_NL5FEDUTqIDecSR_Nm) -> Merge/5
  Equal/1 -> If/1
  Equal4/1 -> If/5
  VTQD_TqTargetShaftSpd_rpm/1 -> [VTQD_TqTargetShaftSpd_rpm]
  [VTQD_RegenMode_enum] -> Equal1/1
  LV2/1(VTQR_NL2FEDUTqDecSR_Nm) -> Merge/2
  If/1 -> LV1/Action
  [VTQD_RegenMode_enum] -> Equal3/1
  [VTQD_TqTargetShaftSpd_rpm] -> OPD/2(VTQD_TqTargetShaftSpd_rpm)
  Constant/1 -> Equal/2
  Merge/1 -> VTQR_NORMALFEDURateLimitDec_Nm/1  "VTQR_NORMALFEDURateLimitDec_Nm"
  Equal1/1 -> If/2
  VTQR_FEDUWhlTqReqSmoothDelay_Nm/1 -> [VTQR_FEDUWhlTqReqSmoothDelay_Nm]
  If/6 -> OPD/Action
  [VTQD_TqTargetShaftSpd_rpm] -> LV3/2(VTQD_TqTargetShaftSpd_rpm)
  Equal3/1 -> If/4
  [VTQR_FEDUWhlTqReqSmoothDelay_Nm] -> LV4/1(VTQR_FEDUWhlTqReqSmoothDelay_Nm)
  If/4 -> LV4/Action
  Constant2/1 -> Equal2/2
  LV3/1(VTQR_NL3FEDUTqDecSR_Nm) -> Merge/3
  LV1/1(VTQR_NL1FEDUTqDecSR_Nm) -> Merge/1
  [VTQR_FEDUWhlTqReqSmoothDelay_Nm] -> LV1/1(VTQR_FEDUWhlTqReqSmoothDelay_Nm)
  [VTQR_FEDUWhlTqReqSmoothDelay_Nm] -> LV2/1(VTQR_FEDUWhlTqReqSmoothDelay_Nm)
  LV4/1(VTQR_NL4FEDUTqDecSR_Nm) -> Merge/4
  [VTQD_RegenMode_enum] -> Equal/1
  [VTQR_FEDUWhlTqReqSmoothDelay_Nm] -> LV3/1(VTQR_FEDUWhlTqReqSmoothDelay_Nm)
  If/2 -> LV2/Action
  If/5 -> LV5/Action
  [VTQR_FEDUWhlTqReqSmoothDelay_Nm] -> OPD/1(VTQR_FEDUWhlTqReqSmoothDelay_Nm)
  [VTQD_TqTargetShaftSpd_rpm] -> LV5/2(VTQD_TqTargetShaftSpd_rpm)
  [VTQD_TqTargetShaftSpd_rpm] -> LV1/2(VTQD_TqTargetShaftSpd_rpm)
  [VTQD_TqTargetShaftSpd_rpm] -> LV4/2(VTQD_TqTargetShaftSpd_rpm)
  [VTQR_FEDUWhlTqReqSmoothDelay_Nm] -> LV5/1(VTQR_FEDUWhlTqReqSmoothDelay_Nm)
  [VTQD_RegenMode_enum] -> Equal2/1
  [VTQD_RegenMode_enum] -> Equal5/1
  Constant5/1 -> Equal5/2
  Constant1/1 -> Equal1/2
  Constant4/1 -> Equal4/2
  VTQD_RegenMode_enum/1 -> [VTQD_RegenMode_enum]
  [VTQD_TqTargetShaftSpd_rpm] -> Invalid/2(VTQD_TqTargetShaftSpd_rpm)
  [VTQR_FEDUWhlTqReqSmoothDelay_Nm] -> Invalid/1(VTQR_FEDUWhlTqReqSmoothDelay_Nm)
  If/7 -> Invalid/Action
  Invalid/1(VTQR_NL1FEDUTqDecSR_Nm) -> Merge/7

== system tqr/TQR/Determine Torque Request/TorqueArbitrament/TorqueSmooth/Front wheel rate limit determination/VTQR_NORMALFEDURateLimitInc_Nm ==
  VDHP_ActAPSPosn_pct : Inport
  VTQD_TqTargetShaftSpd_rpm : Inport  Port=2
  VTQD_RegenMode_enum : Inport  Port=3
  VTQR_FEDUWhlTqReqSmoothDelay_Nm : Inport  Port=4
  Action Port : ActionPort
  Constant : Constant  Value=ENUM_REGENLEVEL_LV1
  Constant1 : Constant  Value=ENUM_REGENLEVEL_LV2
  Constant2 : Constant  Value=ENUM_REGENLEVEL_LV3
  Constant3 : Constant  Value=ENUM_REGENLEVEL_LV4
  Constant4 : Constant  Value=ENUM_REGENLEVEL_LV5
  Constant5 : Constant  Value=ENUM_REGENLEVEL_OPD
  Constant6 : Constant  Value=KTQR_EnNormalFrIncGain_enum
  Constant7 : Constant  Value=ONE_FLOAT
  Equal{,1..5} (6 alike) : RelationalOperator  Operator===  OutDataTypeStr=boolean  RndMeth=Simplest
  If : If  NumInputs=6  IfExpression=u1~= 0  ElseIfExpressions=u2 ~= 0, u3 ~= 0,u4 ~= 0,u5~=0,u6~=0
  Invalid : Subsystem  TreatAsAtomicUnit=on
  LV1 : Subsystem  TreatAsAtomicUnit=on
  LV2 : Subsystem  TreatAsAtomicUnit=on
  LV3 : Subsystem  TreatAsAtomicUnit=on
  LV4 : Subsystem  TreatAsAtomicUnit=on
  LV5 : Subsystem  TreatAsAtomicUnit=on
  MTQR_NormalTqFrIncGain_Z_c : Lookup_n-D  BreakpointsForDimension1=ATQR_NormalTqFrIncGain_Y_pct  BreakpointsForDimension2=ATQR_NormalTqFrIncGain_X_Nm  Table=MTQR_NormalTqFrIncGain_Z_c  ExtrapMethod=Clip  InternalRulePriority=Speed  RndMeth=Simplest  InputSameDT=on
      settings: InputPortMap=u0,u1
  Merge : Merge  Inputs=7
  OPD : Subsystem  TreatAsAtomicUnit=on
  Relational Operator : RelationalOperator  OutDataTypeStr=boolean  RndMeth=Simplest
  Switch : Switch  Criteria=u2 > Threshold
  VTQR_NORMALFEDURateLimitInc_Nm : Outport
  wires:
  VDHP_ActAPSPosn_pct/1 -> [VDHP_ActAPSPosn_pct]
  Merge/1 -> VTQR_NORMALFEDURateLimitInc_Nm/1  "VTQR_NORMALFEDURateLimitInc_Nm"
  VTQD_TqTargetShaftSpd_rpm/1 -> [VTQD_TqTargetShaftSpd_rpm]
  [VTQD_TqTargetShaftSpd_rpm] -> LV3/2(VTQD_TqTargetShaftSpd_rpm)
  LV3/1(VTQR_NL3FEDUTqIncSR_Nm) -> Merge/3
  LV4/1(VTQR_NL4FEDUTqIncSR_Nm) -> Merge/4
  [VTQD_RegenMode_enum] -> Equal1/1
  If/6 -> OPD/Action
  LV1/1(VTQR_NL1FEDUTqIncSR_Nm) -> Merge/1
  If/5 -> LV5/Action
  [VTQD_RegenMode_enum] -> Equal/1
  Constant1/1 -> Equal1/2
  Equal4/1 -> If/5
  Constant5/1 -> Equal5/2
  LV5/1(VTQR_NL5FEDUTqIncSR_Nm) -> Merge/5
  Equal/1 -> If/1
  [VDHP_ActAPSPosn_pct] -> LV4/1(VDHP_ActAPSPosn_pct)
  [VTQD_RegenMode_enum] -> Equal2/1
  [VTQD_TqTargetShaftSpd_rpm] -> LV4/2(VTQD_TqTargetShaftSpd_rpm)
  If/2 -> LV2/Action
  If/3 -> LV3/Action
  [VDHP_ActAPSPosn_pct] -> LV5/1(VDHP_ActAPSPosn_pct)
  [VDHP_ActAPSPosn_pct] -> LV2/1(VDHP_ActAPSPosn_pct)
  Constant3/1 -> Equal3/2
  [VTQD_TqTargetShaftSpd_rpm] -> OPD/2(VTQD_TqTargetShaftSpd_rpm)
  Constant/1 -> Equal/2
  If/4 -> LV4/Action
  [VTQD_RegenMode_enum] -> Equal3/1
  [VDHP_ActAPSPosn_pct] -> LV3/1(VDHP_ActAPSPosn_pct)
  OPD/1(VTQR_NOPDFEDUTqIncSR_Nm) -> Merge/6
  Constant4/1 -> Equal4/2
  [VTQD_TqTargetShaftSpd_rpm] -> LV2/2(VTQD_TqTargetShaftSpd_rpm)
  [VTQD_RegenMode_enum] -> Equal5/1
  Equal2/1 -> If/3
  Constant2/1 -> Equal2/2
  [VTQD_TqTargetShaftSpd_rpm] -> LV1/2(VTQD_TqTargetShaftSpd_rpm)
  Equal3/1 -> If/4
  [VTQD_TqTargetShaftSpd_rpm] -> LV5/2(VTQD_TqTargetShaftSpd_rpm)
  LV2/1(VTQR_NL2FEDUTqIncSR_Nm) -> Merge/2
  Equal5/1 -> If/6
  [VDHP_ActAPSPosn_pct] -> LV1/1(VDHP_ActAPSPosn_pct)
  Equal1/1 -> If/2
  If/1 -> LV1/Action
  [VDHP_ActAPSPosn_pct] -> OPD/1(VDHP_ActAPSPosn_pct)
  [VTQD_RegenMode_enum] -> Equal4/1
  VTQD_RegenMode_enum/1 -> [VTQD_RegenMode_enum]
  [VDHP_ActAPSPosn_pct] -> Invalid/1(VDHP_ActAPSPosn_pct)
  [VTQD_TqTargetShaftSpd_rpm] -> Invalid/2(VTQD_TqTargetShaftSpd_rpm)
  If/7 -> Invalid/Action
  Invalid/1(VTQR_NL1FEDUTqIncSR_Nm) -> Merge/7
  [VTQR_NormalTqFrIncGain_c] -> LV2/3(VTQR_NormalTqFrIncGain_c)
  VTQR_FEDUWhlTqReqSmoothDelay_Nm/1 -> [VTQR_FEDUWhlTqReqSmoothDelay_Nm]
  [VTQR_FEDUWhlTqReqSmoothDelay_Nm] -> MTQR_NormalTqFrIncGain_Z_c/2
  [VDHP_ActAPSPosn_pct] -> MTQR_NormalTqFrIncGain_Z_c/1
  [VTQR_NormalTqFrIncGain_c] -> LV3/3(VTQR_NormalTqFrIncGain_c)
  [VTQD_RegenMode_enum] -> Relational Operator/1
  Constant6/1 -> Relational Operator/2
  Constant7/1 -> Switch/3
  Relational Operator/1 -> Switch/2
  MTQR_NormalTqFrIncGain_Z_c/1 -> Switch/1
  Switch/1 -> [VTQR_NormalTqFrIncGain_c]  "VTQR_NormalTqFrIncGain_c"
  [VTQR_NormalTqFrIncGain_c] -> LV4/3(VTQR_NormalTqFrIncGain_c)
  [VTQR_NormalTqFrIncGain_c] -> LV5/3(VTQR_NormalTqFrIncGain_c)
  [VTQR_NormalTqFrIncGain_c] -> OPD/3(VTQR_NormalTqFrIncGain_c)

== system tqr/TQR/Determine Torque Request/TorqueArbitrament/TorqueSmooth/Front wheel rate limit determination/VTQR_SPORTFEDURateLimitDec_Nm ==
  VTQR_FEDUWhlTqReqSmoothDelay_Nm : Inport
  VTQD_TqTargetShaftSpd_rpm : Inport  Port=2
  VTQD_RegenMode_enum : Inport  Port=3
  Action Port : ActionPort
  Constant : Constant  Value=ENUM_REGENLEVEL_LV1
  Constant1 : Constant  Value=ENUM_REGENLEVEL_LV2
  Constant2 : Constant  Value=ENUM_REGENLEVEL_LV3
  Constant3 : Constant  Value=ENUM_REGENLEVEL_LV4
  Constant4 : Constant  Value=ENUM_REGENLEVEL_LV5
  Constant5 : Constant  Value=ENUM_REGENLEVEL_OPD
  Equal{,1..5} (6 alike) : RelationalOperator  Operator===  OutDataTypeStr=boolean  RndMeth=Simplest
  If : If  NumInputs=6  IfExpression=u1~= 0  ElseIfExpressions=u2 ~= 0, u3 ~= 0,u4 ~= 0,u5~=0,u6~=0
  Invalid : Subsystem  TreatAsAtomicUnit=on
  LV1 : Subsystem  AncestorBlock=tqr/TQR/Determine Torque Request/TorqueArbitrament/TorqueSmooth/Front wheel rate limit determination/VTQR_ECOFEDURateLimitDec_Nm/LV1  TreatAsAtomicUnit=on
  LV2 : Subsystem  AncestorBlock=tqr/TQR/Determine Torque Request/TorqueArbitrament/TorqueSmooth/Front wheel rate limit determination/VTQR_ECOFEDURateLimitDec_Nm/LV2  TreatAsAtomicUnit=on
  LV3 : Subsystem  AncestorBlock=tqr/TQR/Determine Torque Request/TorqueArbitrament/TorqueSmooth/Front wheel rate limit determination/VTQR_ECOFEDURateLimitDec_Nm/LV3  TreatAsAtomicUnit=on
  LV4 : Subsystem  AncestorBlock=tqr/TQR/Determine Torque Request/TorqueArbitrament/TorqueSmooth/Front wheel rate limit determination/VTQR_ECOFEDURateLimitDec_Nm/LV4  TreatAsAtomicUnit=on
  LV5 : Subsystem  AncestorBlock=tqr/TQR/Determine Torque Request/TorqueArbitrament/TorqueSmooth/Front wheel rate limit determination/VTQR_ECOFEDURateLimitDec_Nm/LV5  TreatAsAtomicUnit=on
  Merge : Merge  Inputs=7
  OPD : Subsystem  AncestorBlock=tqr/TQR/Determine Torque Request/TorqueArbitrament/TorqueSmooth/Front wheel rate limit determination/VTQR_ECOFEDURateLimitDec_Nm/OPD  TreatAsAtomicUnit=on
  VTQR_SPORTFEDURateLimitDec_Nm : Outport
  wires:
  If/5 -> LV5/Action
  Constant2/1 -> Equal2/2
  LV5/1(VTQR_SL5FEDUTqIDecSR_Nm) -> Merge/5
  VTQR_FEDUWhlTqReqSmoothDelay_Nm/1 -> [VTQR_FEDUWhlTqReqSmoothDelay_Nm]
  Merge/1 -> VTQR_SPORTFEDURateLimitDec_Nm/1  "VTQR_SPORTFEDURateLimitDec_Nm"
  If/1 -> LV1/Action
  VTQD_TqTargetShaftSpd_rpm/1 -> [VTQD_TqTargetShaftSpd_rpm]
  [VTQR_FEDUWhlTqReqSmoothDelay_Nm] -> LV3/1(VTQR_FEDUWhlTqReqSmoothDelay_Nm)
  LV1/1(VTQR_SL1FEDUTqDecSR_Nm) -> Merge/1
  Constant/1 -> Equal/2
  [VTQD_RegenMode_enum] -> Equal/1
  Constant1/1 -> Equal1/2
  Equal/1 -> If/1
  Equal3/1 -> If/4
  LV4/1(VTQR_SL4FEDUTqDecSR_Nm) -> Merge/4
  [VTQD_RegenMode_enum] -> Equal3/1
  [VTQD_TqTargetShaftSpd_rpm] -> LV5/2(VTQD_TqTargetShaftSpd_rpm)
  [VTQD_TqTargetShaftSpd_rpm] -> LV3/2(VTQD_TqTargetShaftSpd_rpm)
  If/4 -> LV4/Action
  [VTQD_RegenMode_enum] -> Equal1/1
  Equal1/1 -> If/2
  [VTQR_FEDUWhlTqReqSmoothDelay_Nm] -> LV5/1(VTQR_FEDUWhlTqReqSmoothDelay_Nm)
  If/6 -> OPD/Action
  If/2 -> LV2/Action
  Equal4/1 -> If/5
  LV3/1(VTQR_SL3FEDUTqDecSR_Nm) -> Merge/3
  [VTQR_FEDUWhlTqReqSmoothDelay_Nm] -> LV2/1(VTQR_FEDUWhlTqReqSmoothDelay_Nm)
  Equal2/1 -> If/3
  [VTQD_RegenMode_enum] -> Equal5/1
  [VTQD_TqTargetShaftSpd_rpm] -> LV1/2(VTQD_TqTargetShaftSpd_rpm)
  [VTQR_FEDUWhlTqReqSmoothDelay_Nm] -> LV4/1(VTQR_FEDUWhlTqReqSmoothDelay_Nm)
  [VTQR_FEDUWhlTqReqSmoothDelay_Nm] -> LV1/1(VTQR_FEDUWhlTqReqSmoothDelay_Nm)
  [VTQD_RegenMode_enum] -> Equal2/1
  Constant3/1 -> Equal3/2
  [VTQD_TqTargetShaftSpd_rpm] -> LV2/2(VTQD_TqTargetShaftSpd_rpm)
  Constant5/1 -> Equal5/2
  [VTQR_FEDUWhlTqReqSmoothDelay_Nm] -> OPD/1(VTQR_FEDUWhlTqReqSmoothDelay_Nm)
  [VTQD_TqTargetShaftSpd_rpm] -> LV4/2(VTQD_TqTargetShaftSpd_rpm)
  Equal5/1 -> If/6
  OPD/1(VTQR_SOPDFEDUTqDecSR_Nm) -> Merge/6
  Constant4/1 -> Equal4/2
  LV2/1(VTQR_SL2FEDUTqDecSR_Nm) -> Merge/2
  If/3 -> LV3/Action
  [VTQD_RegenMode_enum] -> Equal4/1
  [VTQD_TqTargetShaftSpd_rpm] -> OPD/2(VTQD_TqTargetShaftSpd_rpm)
  VTQD_RegenMode_enum/1 -> [VTQD_RegenMode_enum]
  [VTQR_FEDUWhlTqReqSmoothDelay_Nm] -> Invalid/1(VTQR_FEDUWhlTqReqSmoothDelay_Nm)
  [VTQD_TqTargetShaftSpd_rpm] -> Invalid/2(VTQD_TqTargetShaftSpd_rpm)
  If/7 -> Invalid/Action
  Invalid/1(VTQR_SL1FEDUTqDecSR_Nm) -> Merge/7

== system tqr/TQR/Determine Torque Request/TorqueArbitrament/TorqueSmooth/Front wheel rate limit determination/VTQR_SPORTFEDURateLimitInc_Nm ==
  VDHP_ActAPSPosn_pct : Inport
  VTQD_TqTargetShaftSpd_rpm : Inport  Port=2
  VTQD_RegenMode_enum : Inport  Port=3
  VTQR_REDUWhlTqReqSmoothDelay_Nm : Inport  Port=4
  Action Port : ActionPort
  Constant : Constant  Value=ENUM_REGENLEVEL_LV1
  Constant1 : Constant  Value=ENUM_REGENLEVEL_LV2
  Constant2 : Constant  Value=ENUM_REGENLEVEL_LV3
  Constant3 : Constant  Value=ENUM_REGENLEVEL_LV4
  Constant4 : Constant  Value=ENUM_REGENLEVEL_LV5
  Constant5 : Constant  Value=ENUM_REGENLEVEL_OPD
  Constant6 : Constant  Value=KTQR_EnSportFrIncGain_enum
  Constant7 : Constant  Value=ONE_FLOAT
  Equal{,1..5} (6 alike) : RelationalOperator  Operator===  OutDataTypeStr=boolean  RndMeth=Simplest
  If : If  NumInputs=6  IfExpression=u1~= 0  ElseIfExpressions=u2 ~= 0, u3 ~= 0,u4 ~= 0,u5~=0,u6~=0
  Invalid : Subsystem  TreatAsAtomicUnit=on
  LV1 : Subsystem  TreatAsAtomicUnit=on
  LV2 : Subsystem  AncestorBlock=tqr/TQR/Determine Torque Request/TorqueArbitrament/TorqueSmooth/Front wheel rate limit determination/VTQR_ECOFEDURateLimitInc_Nm/LV2  TreatAsAtomicUnit=on
  LV3 : Subsystem  TreatAsAtomicUnit=on
  LV4 : Subsystem  TreatAsAtomicUnit=on
  LV5 : Subsystem  TreatAsAtomicUnit=on
  MTQR_SportTqFrIncGain_Z_c : Lookup_n-D  BreakpointsForDimension1=ATQR_SportTqFrIncGain_Y_pct  BreakpointsForDimension2=ATQR_SportTqFrIncGain_X_Nm  Table=MTQR_SportTqFrIncGain_Z_c  ExtrapMethod=Clip  InternalRulePriority=Speed  RndMeth=Simplest  InputSameDT=on
      settings: InputPortMap=u0,u1
  Merge : Merge  Inputs=7
  OPD : Subsystem  TreatAsAtomicUnit=on
  Relational Operator : RelationalOperator  OutDataTypeStr=boolean  RndMeth=Simplest
  Switch : Switch  Criteria=u2 > Threshold
  VTQR_SPORTFEDURateLimitInc_Nm : Outport
  wires:
  VDHP_ActAPSPosn_pct/1 -> [VDHP_ActAPSPosn_pct]
  Merge/1 -> VTQR_SPORTFEDURateLimitInc_Nm/1  "VTQR_SPORTFEDURateLimitInc_Nm"
  VTQD_TqTargetShaftSpd_rpm/1 -> [VTQD_TqTargetShaftSpd_rpm]
  [VTQD_TqTargetShaftSpd_rpm] -> LV3/2(VTQD_TqTargetShaftSpd_rpm)
  LV3/1(VTQR_SL3FEDUTqIncSR_Nm) -> Merge/3
  LV4/1(VTQR_SL4FEDUTqIncSR_Nm) -> Merge/4
  [VTQD_RegenMode_enum] -> Equal1/1
  If/6 -> OPD/Action
  LV1/1(VTQR_SL1FEDUTqIncSR_Nm) -> Merge/1
  If/5 -> LV5/Action
  [VTQD_RegenMode_enum] -> Equal/1
  Constant1/1 -> Equal1/2
  Equal4/1 -> If/5
  Constant5/1 -> Equal5/2
  LV5/1(VTQR_SL5FEDUTqIncSR_Nm) -> Merge/5
  Equal/1 -> If/1
  [VDHP_ActAPSPosn_pct] -> LV4/1(VDHP_ActAPSPosn_pct)
  [VTQD_RegenMode_enum] -> Equal2/1
  [VTQD_TqTargetShaftSpd_rpm] -> LV4/2(VTQD_TqTargetShaftSpd_rpm)
  If/2 -> LV2/Action
  If/3 -> LV3/Action
  [VDHP_ActAPSPosn_pct] -> LV5/1(VDHP_ActAPSPosn_pct)
  [VDHP_ActAPSPosn_pct] -> LV2/1(VDHP_ActAPSPosn_pct)
  Constant3/1 -> Equal3/2
  [VTQD_TqTargetShaftSpd_rpm] -> OPD/2(VTQD_TqTargetShaftSpd_rpm)
  Constant/1 -> Equal/2
  If/4 -> LV4/Action
  [VTQD_RegenMode_enum] -> Equal3/1
  [VDHP_ActAPSPosn_pct] -> LV3/1(VDHP_ActAPSPosn_pct)
  OPD/1(VTQR_SOPDFEDUTqIncSR_Nm) -> Merge/6
  Constant4/1 -> Equal4/2
  [VTQD_TqTargetShaftSpd_rpm] -> LV2/2(VTQD_TqTargetShaftSpd_rpm)
  [VTQD_RegenMode_enum] -> Equal5/1
  Equal2/1 -> If/3
  Constant2/1 -> Equal2/2
  [VTQD_TqTargetShaftSpd_rpm] -> LV1/2(VTQD_TqTargetShaftSpd_rpm)
  Equal3/1 -> If/4
  [VTQD_TqTargetShaftSpd_rpm] -> LV5/2(VTQD_TqTargetShaftSpd_rpm)
  LV2/1(VTQR_SL2FEDUTqIncSR_Nm) -> Merge/2
  Equal5/1 -> If/6
  [VDHP_ActAPSPosn_pct] -> LV1/1(VDHP_ActAPSPosn_pct)
  Equal1/1 -> If/2
  If/1 -> LV1/Action
  [VDHP_ActAPSPosn_pct] -> OPD/1(VDHP_ActAPSPosn_pct)
  [VTQD_RegenMode_enum] -> Equal4/1
  VTQD_RegenMode_enum/1 -> [VTQD_RegenMode_enum]
  [VDHP_ActAPSPosn_pct] -> Invalid/1(VDHP_ActAPSPosn_pct)
  [VTQD_TqTargetShaftSpd_rpm] -> Invalid/2(VTQD_TqTargetShaftSpd_rpm)
  If/7 -> Invalid/Action
  Invalid/1(VTQR_SL1FEDUTqIncSR_Nm) -> Merge/7
  [VDHP_ActAPSPosn_pct] -> MTQR_SportTqFrIncGain_Z_c/1
  [VTQR_REDUWhlTqReqSmoothDelay_Nm] -> MTQR_SportTqFrIncGain_Z_c/2
  VTQR_REDUWhlTqReqSmoothDelay_Nm/1 -> [VTQR_REDUWhlTqReqSmoothDelay_Nm]
  [VTQR_SportTqFrIncGain_c] -> LV1/3(VTQR_SportTqFrIncGain_c)
  [VTQR_SportTqFrIncGain_c] -> LV2/3(VTQR_SportTqFrIncGain_c)
  [VTQR_SportTqFrIncGain_c] -> LV3/3(VTQR_SportTqFrIncGain_c)
  [VTQR_SportTqFrIncGain_c] -> LV4/3(VTQR_SportTqFrIncGain_c)
  [VTQR_SportTqFrIncGain_c] -> LV5/3(VTQR_SportTqFrIncGain_c)
  [VTQR_SportTqFrIncGain_c] -> OPD/3(VTQR_SportTqFrIncGain_c)
  Constant6/1 -> Relational Operator/2
  Constant7/1 -> Switch/3
  Relational Operator/1 -> Switch/2
  MTQR_SportTqFrIncGain_Z_c/1 -> Switch/1
  [VTQD_RegenMode_enum] -> Relational Operator/1
  Switch/1 -> [VTQR_SportTqFrIncGain_c]  "VTQR_SportTqFrIncGain_c"

== system tqr/TQR/Determine Torque Request/TorqueArbitrament/TorqueSmooth/Rear First order filter input tau map and determination/VTQR_ECOREDUTs_c ==
  VTQR_FEDUWhlTqReqSmoothDelay_Nm : Inport
  VTQD_TqTargetShaftSpd_rpm : Inport  Port=2
  VTQD_RegenMode_enum : Inport  Port=3
  VTQD_RollRegenEnable_flg : Inport  Port=4
  Action Port : ActionPort
  Constant : Constant  Value=ENUM_REGENLEVEL_LV1
  Constant1 : Constant  Value=ENUM_REGENLEVEL_LV2
  Constant2 : Constant  Value=ENUM_REGENLEVEL_LV3
  Constant3 : Constant  Value=ENUM_REGENLEVEL_LV4
  Constant4 : Constant  Value=ENUM_REGENLEVEL_LV5
  Constant5 : Constant  Value=ENUM_REGENLEVEL_OPD
  Equal{,1..5} (6 alike) : RelationalOperator  Operator===  OutDataTypeStr=boolean  RndMeth=Simplest
  If : If  NumInputs=6  IfExpression=u1~= 0  ElseIfExpressions=u2 ~= 0, u3 ~= 0,u4 ~= 0,u5~=0,u6~=0
  Invalid : Subsystem  TreatAsAtomicUnit=on
  LV1 : Subsystem  AncestorBlock=tqr/TQR/Determine Torque Request/TorqueArbitrament/TorqueSmooth/Front First order filter input tau map and determination/VTQR_NORMALFEDUTs_c/LV1  TreatAsAtomicUnit=on
  LV2 : Subsystem  AncestorBlock=tqr/TQR/Determine Torque Request/TorqueArbitrament/TorqueSmooth/Front First order filter input tau map and determination/VTQR_NORMALFEDUTs_c/LV2  TreatAsAtomicUnit=on
  LV3 : Subsystem  AncestorBlock=tqr/TQR/Determine Torque Request/TorqueArbitrament/TorqueSmooth/Front First order filter input tau map and determination/VTQR_NORMALFEDUTs_c/LV3  TreatAsAtomicUnit=on
  LV4 : Subsystem  AncestorBlock=tqr/TQR/Determine Torque Request/TorqueArbitrament/TorqueSmooth/Front First order filter input tau map and determination/VTQR_NORMALFEDUTs_c/LV4  TreatAsAtomicUnit=on
  LV5 : Subsystem  AncestorBlock=tqr/TQR/Determine Torque Request/TorqueArbitrament/TorqueSmooth/Front First order filter input tau map and determination/VTQR_NORMALFEDUTs_c/LV5  TreatAsAtomicUnit=on
  Merge : Merge  Inputs=7
  OPD : Subsystem  AncestorBlock=tqr/TQR/Determine Torque Request/TorqueArbitrament/TorqueSmooth/Front First order filter input tau map and determination/VTQR_NORMALFEDUTs_c/OPD  TreatAsAtomicUnit=on
  VTQR_ECOREDUTs_c : Outport
  wires:
  LV2/1(VTQR_EL2REDUTs_c) -> Merge/2
  LV4/1(VTQR_EL4REDUTs_c) -> Merge/4
  If/6 -> OPD/Action
  [VTQR_REDUWhlTqReqSmoothDelay_Nm] -> LV1/1(VTQR_REDUWhlTqReqSmoothDelay_Nm)
  Equal4/1 -> If/5
  [VTQD_TqTargetShaftSpd_rpm] -> LV3/2(VTQD_TqTargetShaftSpd_rpm)
  LV1/1(VTQR_EL1REDUTsOrRegen_C) -> Merge/1
  Constant1/1 -> Equal1/2
  [VTQD_RegenMode_enum] -> Equal3/1
  VTQR_FEDUWhlTqReqSmoothDelay_Nm/1 -> [VTQR_REDUWhlTqReqSmoothDelay_Nm]
  Constant5/1 -> Equal5/2
  [VTQD_TqTargetShaftSpd_rpm] -> OPD/2(VTQD_TqTargetShaftSpd_rpm)
  [VTQR_REDUWhlTqReqSmoothDelay_Nm] -> OPD/1(VTQR_FEDUWhlTqReqSmoothDelay_Nm)
  Equal3/1 -> If/4
  LV3/1(VTQR_EL3REDUTs_c) -> Merge/3
  Equal1/1 -> If/2
  VTQD_TqTargetShaftSpd_rpm/1 -> [VTQD_TqTargetShaftSpd_rpm]
  Equal2/1 -> If/3
  [VTQR_REDUWhlTqReqSmoothDelay_Nm] -> LV3/1(VTQR_FEDUWhlTqReqSmoothDelay_Nm)
  VTQD_RegenMode_enum/1 -> [VTQD_RegenMode_enum]
  Equal/1 -> If/1
  [VTQD_TqTargetShaftSpd_rpm] -> LV4/2(VTQD_TqTargetShaftSpd_rpm)
  [VTQR_REDUWhlTqReqSmoothDelay_Nm] -> LV4/1(VTQR_FEDUWhlTqReqSmoothDelay_Nm)
  OPD/1(VTQR_EOPDREDUTs_c) -> Merge/6
  [VTQD_TqTargetShaftSpd_rpm] -> LV1/2(VTQD_TqTargetShaftSpd_rpm)
  Constant/1 -> Equal/2
  [VTQD_TqTargetShaftSpd_rpm] -> LV2/2(VTQD_TqTargetShaftSpd_rpm)
  [VTQR_REDUWhlTqReqSmoothDelay_Nm] -> LV2/1(VTQR_FEDUWhlTqReqSmoothDelay_Nm)
  [VTQD_RegenMode_enum] -> Equal2/1
  [VTQD_RegenMode_enum] -> Equal5/1
  Constant2/1 -> Equal2/2
  [VTQD_RegenMode_enum] -> Equal/1
  [VTQD_RegenMode_enum] -> Equal4/1
  Constant4/1 -> Equal4/2
  Constant3/1 -> Equal3/2
  [VTQD_TqTargetShaftSpd_rpm] -> LV5/2(VTQD_TqTargetShaftSpd_rpm)
  [VTQD_RegenMode_enum] -> Equal1/1
  LV5/1(VTQR_EL5REDUTs_c) -> Merge/5
  Equal5/1 -> If/6
  [VTQR_REDUWhlTqReqSmoothDelay_Nm] -> LV5/1(VTQR_FEDUWhlTqReqSmoothDelay_Nm)
  Merge/1 -> VTQR_ECOREDUTs_c/1  "VTQR_ECOREDUTs_c"
  [VTQD_RollRegenEnable_flg] -> LV1/3(VTQD_RollRegenEnable_flg)
  VTQD_RollRegenEnable_flg/1 -> [VTQD_RollRegenEnable_flg]
  If/1 -> LV1/Action
  If/2 -> LV2/Action
  If/3 -> LV3/Action
  If/4 -> LV4/Action
  If/5 -> LV5/Action
  [VTQD_RollRegenEnable_flg] -> Invalid/3(VTQD_RollRegenEnable_flg)
  [VTQD_TqTargetShaftSpd_rpm] -> Invalid/2(VTQD_TqTargetShaftSpd_rpm)
  [VTQR_REDUWhlTqReqSmoothDelay_Nm] -> Invalid/1(VTQR_REDUWhlTqReqSmoothDelay_Nm)
  If/7 -> Invalid/Action
  Invalid/1(VTQR_EL1REDUTsOrRegen_C) -> Merge/7

== system tqr/TQR/Determine Torque Request/TorqueArbitrament/TorqueSmooth/Rear First order filter input tau map and determination/VTQR_LHMREDUTs_c ==
  VTQR_REDUWhlTqReqSmooth_Nm : Inport
  VTQD_TqTargetShaftSpd_rpm : Inport  Port=2
  Action Port : ActionPort
  MTQR_LHMREDUTs_Z_c : Lookup_n-D  BreakpointsForDimension1=ATQR_NL1REDUTs_Y_Nm  BreakpointsForDimension2=ATQR_NL1FEDUTs_X_rpm  Table=MTQR_LHMREDUTs_Z_c  ExtrapMethod=Clip  InternalRulePriority=Speed  RndMeth=Simplest  InputSameDT=on
      settings: InputPortMap=u0,u1
  VTQR_LHMREDUTs_c : Outport
  wires:
  VTQR_REDUWhlTqReqSmooth_Nm/1 -> MTQR_LHMREDUTs_Z_c/1
  VTQD_TqTargetShaftSpd_rpm/1 -> MTQR_LHMREDUTs_Z_c/2
  MTQR_LHMREDUTs_Z_c/1 -> VTQR_LHMREDUTs_c/1  "VTQR_LHMREDUTs_c"

== system tqr/TQR/Determine Torque Request/TorqueArbitrament/TorqueSmooth/Rear First order filter input tau map and determination/VTQR_NORMALREDUTs_c ==
  VTQR_FEDUWhlTqReqSmoothDelay_Nm : Inport
  VTQD_TqTargetShaftSpd_rpm : Inport  Port=2
  VTQD_RegenMode_enum : Inport  Port=3
  Action Port : ActionPort
  Constant : Constant  Value=ENUM_REGENLEVEL_LV1
  Constant1 : Constant  Value=ENUM_REGENLEVEL_LV2
  Constant2 : Constant  Value=ENUM_REGENLEVEL_LV3
  Constant3 : Constant  Value=ENUM_REGENLEVEL_LV4
  Constant4 : Constant  Value=ENUM_REGENLEVEL_LV5
  Constant5 : Constant  Value=ENUM_REGENLEVEL_OPD
  Equal{,1..5} (6 alike) : RelationalOperator  Operator===  OutDataTypeStr=boolean  RndMeth=Simplest
  If : If  NumInputs=6  IfExpression=u1~= 0  ElseIfExpressions=u2 ~= 0, u3 ~= 0,u4 ~= 0,u5~=0,u6~=0
  Invalid : Subsystem  TreatAsAtomicUnit=on
  LV1 : Subsystem  TreatAsAtomicUnit=on
  LV2 : Subsystem  TreatAsAtomicUnit=on
  LV3 : Subsystem  TreatAsAtomicUnit=on
  LV4 : Subsystem  TreatAsAtomicUnit=on
  LV5 : Subsystem  TreatAsAtomicUnit=on
  Merge : Merge  Inputs=7
  OPD : Subsystem  AncestorBlock=tqr/TQR/Determine Torque Request/TorqueArbitrament/TorqueSmooth/Front First order filter input tau map and determination/VTQR_NORMALFEDUTs_c/LV5  TreatAsAtomicUnit=on
  VTQR_NORMALREDUTs_c : Outport
  wires:
  VTQR_FEDUWhlTqReqSmoothDelay_Nm/1 -> [VTQR_REDUWhlTqReqSmoothDelay_Nm]
  VTQD_TqTargetShaftSpd_rpm/1 -> [VTQD_TqTargetShaftSpd_rpm]
  VTQD_RegenMode_enum/1 -> [VTQD_RegenMode_enum]
  Constant/1 -> Equal/2
  [VTQD_RegenMode_enum] -> Equal/1
  Equal/1 -> If/1
  Equal1/1 -> If/2
  Constant1/1 -> Equal1/2
  [VTQD_RegenMode_enum] -> Equal1/1
  Equal2/1 -> If/3
  Constant2/1 -> Equal2/2
  [VTQD_RegenMode_enum] -> Equal2/1
  Equal3/1 -> If/4
  Constant3/1 -> Equal3/2
  [VTQD_RegenMode_enum] -> Equal3/1
  Equal4/1 -> If/5
  Constant4/1 -> Equal4/2
  [VTQD_RegenMode_enum] -> Equal4/1
  [VTQR_REDUWhlTqReqSmoothDelay_Nm] -> LV1/1(VTQR_REDUWhlTqReqSmoothDelay_Nm)
  [VTQD_TqTargetShaftSpd_rpm] -> LV1/2(VTQD_TqTargetShaftSpd_rpm)
  [VTQR_REDUWhlTqReqSmoothDelay_Nm] -> LV2/1(VTQR_REDUWhlTqReqSmoothDelay_Nm)
  [VTQD_TqTargetShaftSpd_rpm] -> LV2/2(VTQD_TqTargetShaftSpd_rpm)
  [VTQR_REDUWhlTqReqSmoothDelay_Nm] -> LV3/1(VTQR_REDUWhlTqReqSmoothDelay_Nm)
  [VTQD_TqTargetShaftSpd_rpm] -> LV3/2(VTQD_TqTargetShaftSpd_rpm)
  [VTQR_REDUWhlTqReqSmoothDelay_Nm] -> LV4/1(VTQR_REDUWhlTqReqSmoothDelay_Nm)
  [VTQD_TqTargetShaftSpd_rpm] -> LV4/2(VTQD_TqTargetShaftSpd_rpm)
  [VTQR_REDUWhlTqReqSmoothDelay_Nm] -> LV5/1(VTQR_REDUWhlTqReqSmoothDelay_Nm)
  [VTQD_TqTargetShaftSpd_rpm] -> LV5/2(VTQD_TqTargetShaftSpd_rpm)
  LV5/1(VTQR_NL5REDUTs_c) -> Merge/5
  LV4/1(VTQR_NL4REDUTs_c) -> Merge/4
  LV3/1(VTQR_NL3REDUTs_c) -> Merge/3
  LV2/1(VTQR_NL2REDUTs_c) -> Merge/2
  LV1/1(VTQR_NL1REDUTs_c) -> Merge/1
  Equal5/1 -> If/6
  [VTQD_RegenMode_enum] -> Equal5/1
  Constant5/1 -> Equal5/2
  [VTQD_TqTargetShaftSpd_rpm] -> OPD/2(VTQD_TqTargetShaftSpd_rpm)
  [VTQR_REDUWhlTqReqSmoothDelay_Nm] -> OPD/1(VTQR_REDUWhlTqReqSmoothDelay_Nm)
  OPD/1(VTQR_NOPDREDUTs_c) -> Merge/6
  Merge/1 -> VTQR_NORMALREDUTs_c/1  "VTQR_NORMALREDUTs_c"
  If/1 -> LV1/Action
  If/2 -> LV2/Action
  If/3 -> LV3/Action
  If/4 -> LV4/Action
  If/5 -> LV5/Action
  If/6 -> OPD/Action
  [VTQD_TqTargetShaftSpd_rpm] -> Invalid/2(VTQD_TqTargetShaftSpd_rpm)
  [VTQR_REDUWhlTqReqSmoothDelay_Nm] -> Invalid/1(VTQR_REDUWhlTqReqSmoothDelay_Nm)
  If/7 -> Invalid/Action
  Invalid/1(VTQR_NL1REDUTs_c) -> Merge/7

== system tqr/TQR/Determine Torque Request/TorqueArbitrament/TorqueSmooth/Rear First order filter input tau map and determination/VTQR_SPORTREDUTs_c ==
  VTQR_FEDUWhlTqReqSmoothDelay_Nm : Inport
  VTQD_TqTargetShaftSpd_rpm : Inport  Port=2
  VTQD_RegenMode_enum : Inport  Port=3
  Action Port : ActionPort
  Constant : Constant  Value=ENUM_REGENLEVEL_LV1
  Constant1 : Constant  Value=ENUM_REGENLEVEL_LV2
  Constant2 : Constant  Value=ENUM_REGENLEVEL_LV3
  Constant3 : Constant  Value=ENUM_REGENLEVEL_LV4
  Constant4 : Constant  Value=ENUM_REGENLEVEL_LV5
  Constant5 : Constant  Value=ENUM_REGENLEVEL_OPD
  Equal{,1..5} (6 alike) : RelationalOperator  Operator===  OutDataTypeStr=boolean  RndMeth=Simplest
  If : If  NumInputs=6  IfExpression=u1~= 0  ElseIfExpressions=u2 ~= 0, u3 ~= 0,u4 ~= 0,u5~=0,u6~=0
  Invalid : Subsystem  TreatAsAtomicUnit=on
  LV1 : Subsystem  AncestorBlock=tqr/TQR/Determine Torque Request/TorqueArbitrament/TorqueSmooth/Front First order filter input tau map and determination/VTQR_ECOFEDUTs_c/LV1  TreatAsAtomicUnit=on
  LV2 : Subsystem  AncestorBlock=tqr/TQR/Determine Torque Request/TorqueArbitrament/TorqueSmooth/Front First order filter input tau map and determination/VTQR_ECOFEDUTs_c/LV2  TreatAsAtomicUnit=on
  LV3 : Subsystem  AncestorBlock=tqr/TQR/Determine Torque Request/TorqueArbitrament/TorqueSmooth/Front First order filter input tau map and determination/VTQR_ECOFEDUTs_c/LV3  TreatAsAtomicUnit=on
  LV4 : Subsystem  AncestorBlock=tqr/TQR/Determine Torque Request/TorqueArbitrament/TorqueSmooth/Front First order filter input tau map and determination/VTQR_ECOFEDUTs_c/LV4  TreatAsAtomicUnit=on
  LV5 : Subsystem  AncestorBlock=tqr/TQR/Determine Torque Request/TorqueArbitrament/TorqueSmooth/Front First order filter input tau map and determination/VTQR_ECOFEDUTs_c/LV5  TreatAsAtomicUnit=on
  Merge : Merge  Inputs=7
  OPD : Subsystem  AncestorBlock=tqr/TQR/Determine Torque Request/TorqueArbitrament/TorqueSmooth/Front First order filter input tau map and determination/VTQR_ECOFEDUTs_c/OPD  TreatAsAtomicUnit=on
  VTQR_SPORTREDUTs_c : Outport
  wires:
  [VTQD_TqTargetShaftSpd_rpm] -> LV4/2(VTQD_TqTargetShaftSpd_rpm)
  Equal/1 -> If/1
  OPD/1(VTQR_SOPDREDUTs_c) -> Merge/6
  [VTQR_REDUWhlTqReqSmoothDelay_Nm] -> LV4/1(VTQR_REDUWhlTqReqSmoothDelay_Nm)
  [VTQR_REDUWhlTqReqSmoothDelay_Nm] -> OPD/1(VTQR_REDUWhlTqReqSmoothDelay_Nm)
  [VTQD_TqTargetShaftSpd_rpm] -> OPD/2(VTQD_TqTargetShaftSpd_rpm)
  VTQD_RegenMode_enum/1 -> [VTQD_RegenMode_enum]
  Equal3/1 -> If/4
  Equal1/1 -> If/2
  LV3/1(VTQR_SL3REDUTs_c) -> Merge/3
  Equal2/1 -> If/3
  Constant5/1 -> Equal5/2
  Equal4/1 -> If/5
  LV1/1(VTQR_SL1REDUTs_c) -> Merge/1
  [VTQD_TqTargetShaftSpd_rpm] -> LV3/2(VTQD_TqTargetShaftSpd_rpm)
  [VTQR_REDUWhlTqReqSmoothDelay_Nm] -> LV1/1(VTQR_REDUWhlTqReqSmoothDelay_Nm)
  VTQR_FEDUWhlTqReqSmoothDelay_Nm/1 -> [VTQR_REDUWhlTqReqSmoothDelay_Nm]
  Constant1/1 -> Equal1/2
  LV4/1(VTQR_SL4REDUTs_c) -> Merge/4
  [VTQD_RegenMode_enum] -> Equal3/1
  LV2/1(VTQR_SL2REDUTs_c) -> Merge/2
  VTQD_TqTargetShaftSpd_rpm/1 -> [VTQD_TqTargetShaftSpd_rpm]
  [VTQR_REDUWhlTqReqSmoothDelay_Nm] -> LV3/1(VTQR_REDUWhlTqReqSmoothDelay_Nm)
  Constant3/1 -> Equal3/2
  [VTQD_TqTargetShaftSpd_rpm] -> LV5/2(VTQD_TqTargetShaftSpd_rpm)
  [VTQD_RegenMode_enum] -> Equal1/1
  [VTQR_REDUWhlTqReqSmoothDelay_Nm] -> LV5/1(VTQR_REDUWhlTqReqSmoothDelay_Nm)
  Equal5/1 -> If/6
  Constant4/1 -> Equal4/2
  LV5/1(VTQR_SL5REDUTs_c) -> Merge/5
  Constant/1 -> Equal/2
  [VTQD_RegenMode_enum] -> Equal4/1
  Constant2/1 -> Equal2/2
  [VTQD_TqTargetShaftSpd_rpm] -> LV2/2(VTQD_TqTargetShaftSpd_rpm)
  [VTQD_TqTargetShaftSpd_rpm] -> LV1/2(VTQD_TqTargetShaftSpd_rpm)
  [VTQR_REDUWhlTqReqSmoothDelay_Nm] -> LV2/1(VTQR_REDUWhlTqReqSmoothDelay_Nm)
  [VTQD_RegenMode_enum] -> Equal/1
  [VTQD_RegenMode_enum] -> Equal5/1
  [VTQD_RegenMode_enum] -> Equal2/1
  Merge/1 -> VTQR_SPORTREDUTs_c/1  "VTQR_SPORTREDUTs_c"
  If/1 -> LV1/Action
  If/2 -> LV2/Action
  If/3 -> LV3/Action
  If/4 -> LV4/Action
  If/5 -> LV5/Action
  If/6 -> OPD/Action
  [VTQD_TqTargetShaftSpd_rpm] -> Invalid/2(VTQD_TqTargetShaftSpd_rpm)
  [VTQR_REDUWhlTqReqSmoothDelay_Nm] -> Invalid/1(VTQR_REDUWhlTqReqSmoothDelay_Nm)
  If/7 -> Invalid/Action
  Invalid/1(VTQR_SL1REDUTs_c) -> Merge/7

== system tqr/TQR/Determine Torque Request/TorqueArbitrament/TorqueSmooth/Rear Torque zero point transfer boundary map/EcoLow ==
  VTQD_TqTargetShaftSpd_rpm : Inport
  Action Port : ActionPort
  MTQR_RTqZeroTransLowBoundE_Y_Nm : Lookup_n-D  NumberOfTableDimensions=1  BreakpointsForDimension1=ATQR_FTqZeroTransUpBoundN_X_rpm  Table=MTQR_RTqZeroTransLowBoundE_Y_Nm  ExtrapMethod=Clip  InternalRulePriority=Speed  RndMeth=Simplest  InputSameDT=on
  VTQR_RTqZeroTransLowBoundE_Nm : Outport
  wires:
  VTQD_TqTargetShaftSpd_rpm/1 -> MTQR_RTqZeroTransLowBoundE_Y_Nm/1
  MTQR_RTqZeroTransLowBoundE_Y_Nm/1 -> VTQR_RTqZeroTransLowBoundE_Nm/1  "VTQR_RTqZeroTransLowBoundE_Nm"

== system tqr/TQR/Determine Torque Request/TorqueArbitrament/TorqueSmooth/Rear Torque zero point transfer boundary map/EcoUP ==
  VTQD_TqTargetShaftSpd_rpm : Inport
  Action Port : ActionPort
  MTQR_RTqZeroTransUpBoundE_Y_Nm : Lookup_n-D  NumberOfTableDimensions=1  BreakpointsForDimension1=ATQR_FTqZeroTransUpBoundN_X_rpm  Table=MTQR_RTqZeroTransUpBoundE_Y_Nm  ExtrapMethod=Clip  InternalRulePriority=Speed  RndMeth=Simplest  InputSameDT=on
  VTQR_RTqZeroTransUpBoundE_Nm : Outport
  wires:
  MTQR_RTqZeroTransUpBoundE_Y_Nm/1 -> VTQR_RTqZeroTransUpBoundE_Nm/1  "VTQR_RTqZeroTransUpBoundE_Nm"
  VTQD_TqTargetShaftSpd_rpm/1 -> MTQR_RTqZeroTransUpBoundE_Y_Nm/1

== system tqr/TQR/Determine Torque Request/TorqueArbitrament/TorqueSmooth/Rear Torque zero point transfer boundary map/NormalLow ==
  VTQD_TqTargetShaftSpd_rpm : Inport
  Action Port : ActionPort
  MTQR_RTqZeroTransLowBoundN_Y_Nm : Lookup_n-D  NumberOfTableDimensions=1  BreakpointsForDimension1=ATQR_FTqZeroTransUpBoundN_X_rpm  Table=MTQR_RTqZeroTransLowBoundN_Y_Nm  ExtrapMethod=Clip  InternalRulePriority=Speed  RndMeth=Simplest  InputSameDT=on
  VTQR_RTqZeroTransLowBoundN_Nm : Outport
  wires:
  MTQR_RTqZeroTransLowBoundN_Y_Nm/1 -> VTQR_RTqZeroTransLowBoundN_Nm/1  "VTQR_RTqZeroTransLowBoundN_Nm"
  VTQD_TqTargetShaftSpd_rpm/1 -> MTQR_RTqZeroTransLowBoundN_Y_Nm/1
